simulink model "Math_Operations_Lib"  (R2020b)
settings: Solver=FixedStepAuto  StartTime=0.0  StopTime=10.0  RelTol=1e-3
settings Model: Creator=Emiliano  LastModifiedBy=Emiliano
settings OptimizationCC: DefaultParameterBehavior=Inlined  UseDivisionForNetSlopeComputation=on  GainParamInheritBuiltInType=on  UseFloatMulNetSlope=on  InlineInvariantSignals=on  PassReuseOutputArgsAs=Individual arguments  ZeroExternalMemoryAtStartup=off  ZeroInternalMemoryAtStartup=off  NoFixptDivByZeroProtection=on  EfficientFloat2IntCast=on  LifeSpan=1  OptimizeBlockOrder=speed  DifferentSizesBufferReuse=on  EfficientTunableParamExpr=on
settings DebuggingCC: ParameterTunabilityLossMsg=error
settings HardwareCC: ProdLongLongMode=on
settings SFSimCC: MATLABDynamicMemAlloc=off
settings RTWCC: Description=Embedded Coder  SystemTargetFile=ert.tlc  TemplateMakefile=ert_default_tmf
settings CodeAppCC: ForceParamTrailComments=on  IgnoreCustomStorageClasses=off  OperatorAnnotations=on  SimulinkDataObjDesc=on  SFDataObjDesc=on  CustomSymbolStrGlobalVar=rt$N$M  CustomSymbolStrType=$N$M  CustomSymbolStrFcn=$N$M$F  CustomSymbolStrMacro=$N$M  InsertBlockDesc=on
settings ERTTargetCC: TargetLangStandard=C99 (ISO)  GenerateSampleERTMain=on  IncludeMdlTerminateFcn=off  CombineSignalStateStructs=on  SuppressErrorStatus=on  SupportAbsoluteTime=off  SupportComplex=off  InlinedParameterPlacement=NonHierarchical  ERTCustomFileTemplate=example_file_process.tlc  ERTFilePackagingFormat=CompactWithDataFile

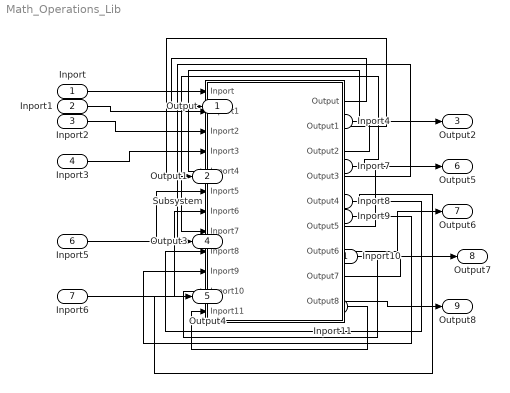
== system Math_Operations_Lib ==
  Inport : Inport
  Inport1 : Inport  Port=2
  Inport2 : Inport  Port=3
  Inport3 : Inport  Port=4
  Inport4 : Inport  Port=5
  Inport5 : Inport  Port=6
  Inport6 : Inport  Port=7
  Inport7 : Inport  Port=8
  Inport8 : Inport  Port=9
  Inport9 : Inport  Port=10
  Inport10 : Inport  Port=11
  Inport11 : Inport  Port=12
  Subsystem : Subsystem
  Output : Outport
  Output1 : Outport  Port=2
  Output2 : Outport  Port=3
  Output3 : Outport  Port=4
  Output4 : Outport  Port=5
  Output5 : Outport  Port=6
  Output6 : Outport  Port=7
  Output7 : Outport  Port=8
  Output8 : Outport  Port=9
  wires:
  Inport/1 -> Subsystem/1(Inport)
  Inport1/1 -> Subsystem/2(Inport1)
  Inport2/1 -> Subsystem/3(Inport2)
  Inport3/1 -> Subsystem/4(Inport3)
  Inport4/1 -> Subsystem/5(Inport4)
  Inport5/1 -> Subsystem/6(Inport5)
  Inport6/1 -> Subsystem/7(Inport6)
  Inport7/1 -> Subsystem/8(Inport7)
  Inport8/1 -> Subsystem/9(Inport8)
  Inport9/1 -> Subsystem/10(Inport9)
  Inport10/1 -> Subsystem/11(Inport10)
  Inport11/1 -> Subsystem/12(Inport11)
  Subsystem/1(Output) -> Output/1
  Subsystem/2(Output1) -> Output1/1
  Subsystem/3(Output2) -> Output2/1
  Subsystem/4(Output3) -> Output3/1
  Subsystem/5(Output4) -> Output4/1
  Subsystem/6(Output5) -> Output5/1
  Subsystem/7(Output6) -> Output6/1
  Subsystem/8(Output7) -> Output7/1
  Subsystem/9(Output8) -> Output8/1

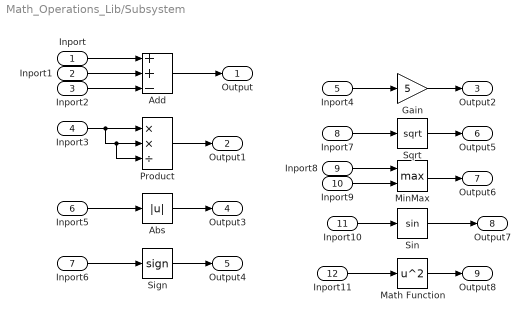
== system Math_Operations_Lib/Subsystem ==
  Inport : Inport
  Inport1 : Inport  Port=2
  Inport2 : Inport  Port=3
  Inport3 : Inport  Port=4
  Inport4 : Inport  Port=5
  Inport5 : Inport  Port=6
  Inport6 : Inport  Port=7
  Inport7 : Inport  Port=8
  Inport8 : Inport  Port=9
  Inport9 : Inport  Port=10
  Inport10 : Inport  Port=11
  Inport11 : Inport  Port=12
  Abs : Abs
  Add : Sum  Inputs=++-
  Gain : Gain  Gain=5
  Math Function : Math  Operator=square  SaturateOnIntegerOverflow=on
  MinMax : MinMax  Function=max  Inputs=2
  Product : Product  Inputs=**/
  Sign : Signum
  Sin : Trigonometry
  Sqrt : Sqrt  SaturateOnIntegerOverflow=on
  Output : Outport
  Output1 : Outport  Port=2
  Output2 : Outport  Port=3
  Output3 : Outport  Port=4
  Output4 : Outport  Port=5
  Output5 : Outport  Port=6
  Output6 : Outport  Port=7
  Output7 : Outport  Port=8
  Output8 : Outport  Port=9
  wires:
  Inport8/1 -> MinMax/1
  Inport4/1 -> Gain/1
  MinMax/1 -> Output6/1
  Inport5/1 -> Abs/1
  Sign/1 -> Output4/1
  Inport6/1 -> Sign/1
  Inport3/1 -> Product/3, Product/2, Product/1
  Inport/1 -> Add/1
  Gain/1 -> Output2/1
  Product/1 -> Output1/1
  Inport1/1 -> Add/2
  Inport2/1 -> Add/3
  Inport7/1 -> Sqrt/1
  Inport10/1 -> Sin/1
  Add/1 -> Output/1
  Abs/1 -> Output3/1
  Sqrt/1 -> Output5/1
  Inport9/1 -> MinMax/2
  Sin/1 -> Output7/1
  Math Function/1 -> Output8/1
  Inport11/1 -> Math Function/1
